simulink model "StanzaSemplice"  (R2022b)
settings: Solver=VariableStepAuto  StartTime=0.0  StopTime=100  RelTol=1e-3
values from neighbouring files (symbols this model uses):
  C = [1]    [StanzaSempliceValues.m]
  Q = 50    [StanzaSempliceValues.m]
  R = 2    [StanzaSempliceValues.m]
  Ta = 10    [StanzaSempliceValues.m]
settings Model: Creator=giuli  LastModifiedBy=giuli

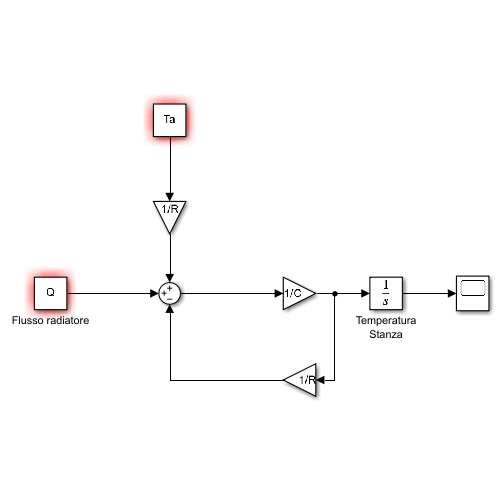
[thumbnail: Simulink's stored preview of the top-level diagram]
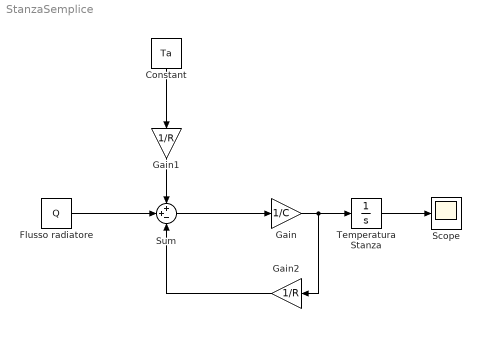
== system StanzaSemplice ==
  Constant : Constant  Value=Ta
  Flusso radiatore : Constant  Value=Q
  Gain : Gain  Gain=1/C
  Gain1 : Gain  Gain=1/R
  Gain2 : Gain  Gain=1/R
  Scope : Scope
  Sum : Sum  Inputs=++-
  Temperatura Stanza : Integrator
  wires:
  Gain/1 -> Gain2/1, Temperatura Stanza/1
  Sum/1 -> Gain/1
  Gain1/1 -> Sum/1
  Constant/1 -> Gain1/1
  Flusso radiatore/1 -> Sum/2
  Gain2/1 -> Sum/3
  Temperatura Stanza/1 -> Scope/1
